simulink model "Control_try_final_2020b"  (R2020b)
settings: Solver=VariableStepAuto  StartTime=0.0  StopTime=inf  RelTol=1e-3
undefined symbols (not defined in the file or in its folder): DiscIntNeverNeededParam
libraries: mobileRoboticsLib x25
(part 7 of 7)

== stateflow chart Control_try_final_2020b/Team_1_behaviour/T1R3 (defender 1)/Team 1 Behaviour/Velocity_Decider ==
  state Robot_Far
    du:
    velocity = 1;
    kick = 0;
  state Robot_Close
    du:
    velocity = 0;
    kick = 1;
  (default) -> Robot_Far
  Robot_Far -> Robot_Close : [DBR <= 0.25]
  Robot_Close -> Robot_Far : [DBR > 0.25]
  data: kick output; DBR input; velocity output

== stateflow chart Control_try_final_2020b/Team_1_behaviour/T1R3 (defender 1)/Team 1 Behaviour/kick_direction/Chart1 ==
  state x_pos
    du:
    Vx = 1
  state x_neg
    du:
    Vx = -1
  (default) -> x_pos
  x_pos -> x_neg : [x > 0]
  x_neg -> x_pos : [x<1]
  data: Vx output; x input

== stateflow chart Control_try_final_2020b/Team_1_behaviour/T1R3 (defender 1)/Team 1 Behaviour/kick_direction/Chart2 ==
  state y_pos
    du:
    Vy = 1
  state y_neg
    du:
    Vy = -1
  (default) -> y_pos
  y_pos -> y_neg : [y > 0]
  y_neg -> y_pos : [y<1]
  data: y input; Vy output

== stateflow chart Control_try_final_2020b/Team_1_behaviour/T1R3 (Defender 2)/Team 1 Behaviour1/Chart4 ==
  state stop
    du:
    w = 0;
    v=0.25 * velocity;
  state RCW
    du:
    w = -1*1;
    v=0;
  state RCCW
    du:
    w =1*1;
    v=0;
  (default) -> stop
  stop -> RCCW [order 2] : [after(1,sec) && DT > 0]
  stop -> RCW [order 1] : [after(1,sec) && DT < 0]
  RCW -> stop [order 1] : [DT<= 0.1 && DT>= -0.1]
  RCCW -> stop [order 1] : [DT<= 0.1 && DT>= -0.1]
  RCCW -> RCW [order 2] : [DT>0]
  RCW -> RCCW [order 2] : [DT<0]
  data: velocity input; v output; DT input; w output

== matlab function Control_try_final_2020b/Team_1_behaviour/T1R3 (Defender 2)/Team 1 Behaviour1/MATLAB Function ==
  data: F input; dF output; dis input; dT input
function dF = fcn(F,dis,dT)


F_x_max = max(abs(F(:,1))) ;
% F_y_max = max(abs(F(:,2))) ;

Fmax = sqrt((F_x_max^2)) ;

fc = sqrt(2*dis*dis*dT) ;

if fc <= Fmax
    dF = fc ;
else
    dF = Fmax ;
end

end

== matlab function Control_try_final_2020b/Team_1_behaviour/T1R3 (Defender 2)/Team 1 Behaviour1/MATLAB Function1 ==
  data: beh input; y output; goal input; team input; rob_loc input; rob_loc1 input; z output
function [y, z] = fcn(beh,goal,team,rob_loc,rob_loc1)
if (beh == 3)
    y = goal;
    z = [10,4];
elseif (beh == 2)
    y = 0.25;
    z = [10,4];
else
    y = team;
    z = [rob_loc1(1), rob_loc1(2)];
end

== stateflow chart Control_try_final_2020b/Team_1_behaviour/T1R3 (defender 1)/Team 1 Behaviour1/Chart1 ==
  state second_coordinate
    du:
    actual_angle = -pi +angle + angle_bot;
  state first_coordinate
    du:
    actual_angle = angle_bot - angle;
  state ffourth_coordinate
    du:
    actual_angle = -(2*pi) + angle + angle_bot
  state Third_coordinate
    du:
    actual_angle =-(pi) - angle + angle_bot;
  (default) -> first_coordinate
  first_coordinate -> second_coordinate [order 1] : [ Rx>Bx && Ry<By ]
  second_coordinate -> first_coordinate [order 1] : [ Rx<Bx && Ry<By]
  ffourth_coordinate -> second_coordinate [order 1] : [ Rx>Bx && Ry<By ]
  first_coordinate -> Third_coordinate [order 3] : [ Rx>Bx && Ry>By]
  second_coordinate -> Third_coordinate [order 3] : [ Rx>Bx && Ry>By ]
  Third_coordinate -> second_coordinate [order 1] : [ Rx>Bx && Ry<By ]
  second_coordinate -> ffourth_coordinate [order 2] : [ Rx<Bx && Ry>By ]
  Third_coordinate -> first_coordinate [order 2] : [ Rx<Bx && Ry<By ]
  ffourth_coordinate -> first_coordinate [order 2] : [ Rx<Bx && Ry<By ]
  first_coordinate -> ffourth_coordinate [order 2] : [ Rx<Bx && Ry>By ]
  Third_coordinate -> ffourth_coordinate [order 3] : [ Rx<Bx && Ry>By ]
  ffourth_coordinate -> Third_coordinate [order 3] : [ Rx>Bx && Ry>By]
  data: Bx input; By input; Rx input; Ry input; angle input; actual_angle output; angle_bot input

== stateflow chart Control_try_final_2020b/Team_1_behaviour/T1R3 (defender 1)/Team 1 Behaviour1/Chart2 ==
  state go_to_ball
    du:
    kick = 0;
    pass_beh = 0;
    if(distance_to_ball < 0.25)
    pass_beh = pass_behaviour_controller(distance_to_goal,nearest_op,nearest_team);
    i = 0;
    else
    velocity = 0.44;
    end
  state pass
    du:
    velocity = 0;
    kick = 1;
  state shoot
    du:
    velocity = 0;
    kick = 1;
  state dribble
    du:
    velocity = 0;
    kick = 1;
  (default) -> go_to_ball
  go_to_ball -> pass [order 1] : [pass_beh == 1&& distance_to_ball < 0.25 ]
  dribble -> go_to_ball : [kick == 1]
  go_to_ball -> dribble [order 3] : [pass_beh == 2 && distance_to_ball < 0.25 ]
  pass -> go_to_ball : [kick == 1]
  go_to_ball -> shoot [order 2] : [pass_beh == 3 && distance_to_ball < 0.25 ]
  shoot -> go_to_ball : [kick == 1]
  data: distancetogoal function_input; nearest_oponent_distance function_input; nearest_team_player_distance function_input; pass_behaviour function_output; kick output =0; distance_to_ball input; velocity output; nearest_team input; nearest_op input; distance_to_goal input; pass_beh output =0; i local =1
  function pass_behaviour  = pass_behaviour_controller(distancetogoal,nearest_oponent_distance,nearest_team_player_distance):
    | function pass_behaviour  = pass_behaviour_controller(distancetogoal,nearest_oponent_distance,nearest_team_player_distance)
    | %PASS_BEHAVIOR Summary of this function goes here
    | %   Detailed explanation goes here
    | behaviourFuzzyFile= getFISCodeGenerationData('pass_behaviour.fis');
    | b = evalfis(behaviourFuzzyFile,[distancetogoal,nearest_oponent_distance,nearest_team_player_distance]);
    | 
    | if ( b<0.4 )
    | pass_behaviour=1;
    | elseif ( 0.4<=b && b<0.6 )
    | pass_behaviour=2;
    | else
    | pass_behaviour=3;
    | end
    | 
    | end

== stateflow chart Control_try_final_2020b/Team_1_behaviour/T1R3 (defender 1)/Team 1 Behaviour1/Chart4 ==
  state stop
    du:
    w = 0;
    v=0.25 * velocity;
  state RCW
    du:
    w = -1*1;
    v=0;
  state RCCW
    du:
    w =1*1;
    v=0;
  (default) -> stop
  stop -> RCCW [order 2] : [after(1,sec) && DT > 0]
  stop -> RCW [order 1] : [after(1,sec) && DT < 0]
  RCW -> stop [order 1] : [DT<= 0.1 && DT>= -0.1]
  RCCW -> stop [order 1] : [DT<= 0.1 && DT>= -0.1]
  RCCW -> RCW [order 2] : [DT>0]
  RCW -> RCCW [order 2] : [DT<0]
  data: velocity input; v output; DT input; w output

== stateflow chart Control_try_final_2020b/Team_2_Behaviour/T2_R1(Goal_Keeper)/control ==
  state Ball_Following
    du:
    kick = 0;
    if (R1_loc_Y>2.7 && R1_loc_Y<5.3)
    if(Ball_loc_Y > R1_loc_Y)
    R1_vel_Y = -0.1;
    elseif (Ball_loc_Y < R1_loc_Y)
    R1_vel_Y = 0.1;
    end
    elseif ( R1_loc_Y > 5.3)
    R1_vel_Y = 0.1;
    elseif ( R1_loc_Y < 2.7)
    R1_vel_Y = -0.1;
    end
    end
  state Ball_Held
    du:
    kick = 1;
  (default) -> Ball_Following
  Ball_Following -> Ball_Held : [GB_dist < 0.25]
  Ball_Held -> Ball_Following : [GB_dist > 0.25]
  data: kick output; R1_loc_X input; Ball_loc_X input; GB_dist input; R1_loc_Y input; Ball_loc_Y input; R1_vel_Y output

== matlab function Control_try_final_2020b/Team_1_behaviour/T1R3 (defender 1)/Team 1 Behaviour1/MATLAB Function ==
  data: F input; dF output; dis input; dT input
function dF = fcn(F,dis,dT)


F_x_max = max(abs(F(:,1))) ;
% F_y_max = max(abs(F(:,2))) ;

Fmax = sqrt((F_x_max^2)) ;

fc = sqrt(2*dis*dis*dT) ;

if fc <= Fmax
    dF = fc ;
else
    dF = Fmax ;
end

end

== stateflow chart Control_try_final_2020b/Team_2_Behaviour/T2_R3(Attacker 1)/Team 1 Behaviour1/Chart2 ==
  state second_coordinate
    du:
    actual_angle = -pi +angle + angle_bot;
  state first_coordinate
    du:
    actual_angle = angle_bot - angle;
  state ffourth_coordinate
    du:
    actual_angle = -(2*pi) + angle + angle_bot
  state Third_coordinate
    du:
    actual_angle =-(pi) - angle + angle_bot;
  (default) -> first_coordinate
  first_coordinate -> second_coordinate [order 1] : [ Rx>Bx && Ry<By ]
  second_coordinate -> first_coordinate [order 1] : [ Rx<Bx && Ry<By]
  ffourth_coordinate -> second_coordinate [order 1] : [ Rx>Bx && Ry<By ]
  first_coordinate -> Third_coordinate [order 3] : [ Rx>Bx && Ry>By]
  second_coordinate -> Third_coordinate [order 3] : [ Rx>Bx && Ry>By ]
  Third_coordinate -> second_coordinate [order 1] : [ Rx>Bx && Ry<By ]
  second_coordinate -> ffourth_coordinate [order 2] : [ Rx<Bx && Ry>By ]
  Third_coordinate -> first_coordinate [order 2] : [ Rx<Bx && Ry<By ]
  ffourth_coordinate -> first_coordinate [order 2] : [ Rx<Bx && Ry<By ]
  first_coordinate -> ffourth_coordinate [order 2] : [ Rx<Bx && Ry>By ]
  Third_coordinate -> ffourth_coordinate [order 3] : [ Rx<Bx && Ry>By ]
  ffourth_coordinate -> Third_coordinate [order 3] : [ Rx>Bx && Ry>By]
  data: Bx input; By input; Rx input; Ry input; angle input; actual_angle output; angle_bot input

== matlab function Control_try_final_2020b/Team_1_behaviour/T1R3 (defender 1)/Team 1 Behaviour1/MATLAB Function1 ==
  data: beh input; y output; goal input; team input; rob_loc input; rob_loc1 input; z output
function [y, z] = fcn(beh,goal,team,rob_loc,rob_loc1)
if (beh == 3)
    y = goal;
    z = [10,4];
elseif (beh == 2)
    y = 0.25;
    z = [10,4];
else
    y = team;
    z = [rob_loc1(1), rob_loc1(2)];
end

== stateflow chart Control_try_final_2020b/Team_2_Behaviour/T2_R1(Goal_Keeper)/min_Distance_Finder/Kick_prob_calc ==
  state bot_2
    du:
    kick_direction = R_2_loc
  state bot_3
    du:
    kick_direction = R_3_loc
  state bot_4
    du:
    kick_direction = R_4_loc
  (default) -> bot_2
  bot_2 -> bot_3 [order 1] : [R1_R3_dis < R1_R2_dis && R1_R3_dis < R1_R4_dis]
  bot_3 -> bot_2 [order 1] : [R1_R2_dis < R1_R3_dis && R1_R2_dis < R1_R4_dis]
  bot_4 -> bot_2 [order 2] : [R1_R2_dis < R1_R3_dis && R1_R2_dis < R1_R4_dis]
  bot_2 -> bot_4 [order 2] : [R1_R4_dis < R1_R3_dis && R1_R4_dis < R1_R2_dis]
  bot_3 -> bot_4 [order 2] : [R1_R4_dis < R1_R3_dis && R1_R4_dis < R1_R2_dis]
  bot_4 -> bot_3 [order 1] : [R1_R3_dis < R1_R2_dis && R1_R3_dis < R1_R4_dis]
  data: R_4_loc input; R_2_loc input; R_3_loc input; R1_R2_dis input; R1_R3_dis input; R1_R4_dis input; kick_direction output

== stateflow chart Control_try_final_2020b/Team_2_Behaviour/T2_R1(Goal_Keeper)/min_Distance_Finder/R2_O_dist_val/Chart ==
  state calculate
    en:
    dist = 0;
    pos_x = 0;
    pos_y =0;
    dist_x =0;
    dist_y = 0;
    i=0;
    du:
    dist = 0;
    for i=1:7
    if (sen_1_val(i,3) > 4)
    pos_x = R_1_loc(1) + sen_1_val(i,1);
    pos_y = R_1_loc(2) + sen_1_val(i,2);
    dist_x = R_2_loc(1) - pos_x;
    dist_y = R_2_loc(2) - pos_y;
    dist = dist + sqrt((dist_x*dist_x) + (dist_y*dist_y));
    end
    end
  (default) -> calculate
  data: R_1_loc input; sen_1_val input; dist output; R_2_loc input; dist_y local; i local; pos_x local; pos_y local; dist_x local

== stateflow chart Control_try_final_2020b/Team_2_Behaviour/T2_R1(Goal_Keeper)/min_Distance_Finder/R3_O_dist_val/Chart ==
  state calculate
    en:
    dist = 0;
    pos_x = 0;
    pos_y =0;
    dist_x =0;
    dist_y = 0;
    i=0;
    du:
    dist = 0;
    for i=1:7
    if (sen_1_val(i,3) > 4)
    pos_x = R_1_loc(1) + sen_1_val(i,1);
    pos_y = R_1_loc(2) + sen_1_val(i,2);
    dist_x = R_2_loc(1) - pos_x;
    dist_y = R_2_loc(2) - pos_y;
    dist = dist + sqrt((dist_x*dist_x) + (dist_y*dist_y));
    end
    end
  (default) -> calculate
  data: R_1_loc input; sen_1_val input; dist output; R_2_loc input; dist_y local; i local; pos_x local; pos_y local; dist_x local

== stateflow chart Control_try_final_2020b/Team_2_Behaviour/T2_R1(Goal_Keeper)/min_Distance_Finder/R4_O_dist_val/Chart ==
  state calculate
    en:
    dist = 0;
    pos_x = 0;
    pos_y =0;
    dist_x =0;
    dist_y = 0;
    i=0;
    du:
    dist = 0;
    for i=1:7
    if (sen_1_val(i,3) > 4)
    pos_x = R_1_loc(1) + sen_1_val(i,1);
    pos_y = R_1_loc(2) + sen_1_val(i,2);
    dist_x = R_2_loc(1) - pos_x;
    dist_y = R_2_loc(2) - pos_y;
    dist = dist + sqrt((dist_x*dist_x) + (dist_y*dist_y));
    end
    end
  (default) -> calculate
  data: R_1_loc input; sen_1_val input; dist output; R_2_loc input; dist_y local; i local; pos_x local; pos_y local; dist_x local

== matlab function Control_try_final_2020b/Team_2_Behaviour/T2_R1(Goal_Keeper)/min_Distance_Finder/zero_padding ==
  data: u input; y output
function y = pad(u)
% Zero-pads object detections to work with arrays of buses

y = zeros(7,3);
numElems = min(size(u,1),7);
for idx = 1:numElems
   y(idx,1:3) = u(idx,1:3); 
end
end

== matlab function Control_try_final_2020b/Team_1_behaviour/T1R3 (defender 1)/Team 1 Behaviour1/MATLAB Function2 ==
  data: u input; y output; r3 input; r4 input
function y = fcn(u , r3, r4)
if u == 4
   y = [r3(1), r3(2)];
else
    y = [r4(1) , r4(2)];
end

== matlab function Control_try_final_2020b/Team_1_behaviour/T1R3 (defender 1)/Team 1 Behaviour1/MATLAB Function3 ==
  data: distance_to_goal1 input; centroid output; goal_keeperY input; distance_to_goal2 input
function centroid  = shooting_spot_rev1_controller(distance_to_goal1, goal_keeperY, distance_to_goal2)
%UNTITLED3 Summary of this function goes here
%   Detailed explanation goes here
ShootingSpotFuzzyFile= getFISCodeGenerationData('shooting_spot_rev1');
C = evalfis(ShootingSpotFuzzyFile,[distance_to_goal1, goal_keeperY, distance_to_goal2]);
if ( C<1 )
% shooting_region=1;
centroid = [10,4.65];
elseif ( 1<=C && C<2 )
% shooting_region=2;
centroid = [10,3.35];
elseif ( 2<=C && C<3 )
% shooting_region=3;
centroid = [10,4.65];
else
% shooting_region=4;
centroid = [10,4.65];
end
end

== matlab function Control_try_final_2020b/Team_1_behaviour/T1R3 (defender 1)/Team 1 Behaviour1/MATLAB Function4 ==
  data: u input; y output
function y = fcn(u)
if u == 3
    y =1;
else 
    y = 0;
end
end

== stateflow chart Control_try_final_2020b/Team_1_behaviour/T1R3 (defender 1)/Team 1 Behaviour1/kick_direction1/Chart1 ==
  state x_pos
    du:
    Vx = 1
  state x_neg
    du:
    Vx = -1
  (default) -> x_pos
  x_pos -> x_neg : [x > 0]
  x_neg -> x_pos : [x<1]
  data: Vx output; x input

== stateflow chart Control_try_final_2020b/Team_1_behaviour/T1R3 (defender 1)/Team 1 Behaviour1/kick_direction1/Chart2 ==
  state y_pos
    du:
    Vy = 1
  state y_neg
    du:
    Vy = -1
  (default) -> y_pos
  y_pos -> y_neg : [y > 0]
  y_neg -> y_pos : [y<1]
  data: y input; Vy output

== matlab function Control_try_final_2020b/Team_1_behaviour/T1R3 (defender 1)/Team 1 Behaviour1/min_Distance_Finder/MATLAB Function ==
  data: min input; y output; rob3 input
function y = fcn(min, rob3)
 if min == rob3
y = 4;
 else 
     y =2;
 end
end

== stateflow chart Control_try_final_2020b/Team_1_behaviour/T1R3 (defender 1)/Team 1 Behaviour1/min_Distance_Finder/R2_O_dist_val/Chart ==
  state calculate
    en:
    dist = 0;
    pos_x = 0;
    pos_y =0;
    dist_x =0;
    dist_y = 0;
    i=0;
    du:
    dist = 0;
    for i=1:7
    if (sen_1_val(i,3) > 4)
    pos_x = R_1_loc(1) + sen_1_val(i,1);
    pos_y = R_1_loc(2) + sen_1_val(i,2);
    dist_x = R_2_loc(1) - pos_x;
    dist_y = R_2_loc(2) - pos_y;
    dist = dist + sqrt((dist_x*dist_x) + (dist_y*dist_y));
    end
    end
  (default) -> calculate
  data: R_1_loc input; sen_1_val input; dist output; R_2_loc input; dist_y local; i local; pos_x local; pos_y local; dist_x local

== stateflow chart Control_try_final_2020b/Team_1_behaviour/T1R3 (defender 1)/Team 1 Behaviour1/min_Distance_Finder/R3_O_dist_val/Chart ==
  state calculate
    en:
    dist = 0;
    pos_x = 0;
    pos_y =0;
    dist_x =0;
    dist_y = 0;
    i=0;
    du:
    dist = 0;
    for i=1:7
    if (sen_1_val(i,3) > 4)
    pos_x = R_1_loc(1) + sen_1_val(i,1);
    pos_y = R_1_loc(2) + sen_1_val(i,2);
    dist_x = R_2_loc(1) - pos_x;
    dist_y = R_2_loc(2) - pos_y;
    dist = dist + sqrt((dist_x*dist_x) + (dist_y*dist_y));
    end
    end
  (default) -> calculate
  data: R_1_loc input; sen_1_val input; dist output; R_2_loc input; dist_y local; i local; pos_x local; pos_y local; dist_x local

== stateflow chart Control_try_final_2020b/Team_1_behaviour/T1R3 (defender 1)/Team 1 Behaviour1/min_Distance_Finder/R4_O_dist_val/Chart ==
  state calculate
    en:
    dist = 0;
    pos_x = 0;
    pos_y =0;
    dist_x =0;
    dist_y = 0;
    i=0;
    du:
    dist = 0;
    for i=1:7
    if (sen_1_val(i,3) > 4)
    pos_x = R_1_loc(1) + sen_1_val(i,1);
    pos_y = R_1_loc(2) + sen_1_val(i,2);
    dist_x = R_2_loc(1) - pos_x;
    dist_y = R_2_loc(2) - pos_y;
    dist = dist + sqrt((dist_x*dist_x) + (dist_y*dist_y));
    end
    end
  (default) -> calculate
  data: R_1_loc input; sen_1_val input; dist output; R_2_loc input; dist_y local; i local; pos_x local; pos_y local; dist_x local
